simulink model "H_inf_2021"  (R2021b)
settings: Solver=VariableStepAuto  StartTime=0.0  StopTime=20  FixedStep=0.01  RelTol=1e-3
values from neighbouring files (symbols this model uses):
  Ask = [0 1 0 0 ... (first row only)    [H_inf_ctrl.m]    (also in H_inf_ctrl_11_2_p.m; H_inf_ctrl_11_3_heavy.m; H_inf_ctrl_11_3_light.m)
  Bsk = [0 0 0 0 ... (first row only)    [H_inf_ctrl.m]    (also in H_inf_ctrl_11_2_p.m; H_inf_ctrl_11_3_heavy.m; H_inf_ctrl_11_3_light.m)
  Csk = [0 1 0 0 ... (first row only)    [H_inf_ctrl.m]    (also in H_inf_ctrl_11_2_p.m; H_inf_ctrl_11_3_heavy.m; H_inf_ctrl_11_3_light.m)
  Dsk = zeros(2,4)    [H_inf_ctrl.m]    (also in H_inf_ctrl_11_2_p.m; H_inf_ctrl_11_3_heavy.m; H_inf_ctrl_11_3_light.m)
undefined symbols (not defined in the file or in its folder): Ainf, Binf, Cinf, Dinf, sigbuilder_block
settings Model: Creator=tawsiful  LastModifiedBy=rivaa
settings DebuggingCC: UnconnectedInputMsg=none  UnconnectedOutputMsg=none  UnconnectedLineMsg=none
settings RTWCC: DLArmComputeVersion=20.02.1

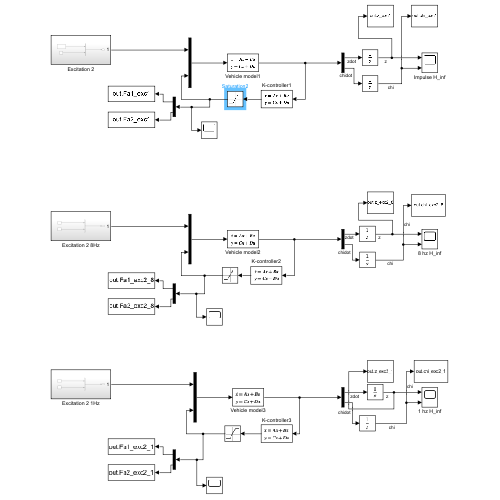
[thumbnail: Simulink's stored preview of the top-level diagram]
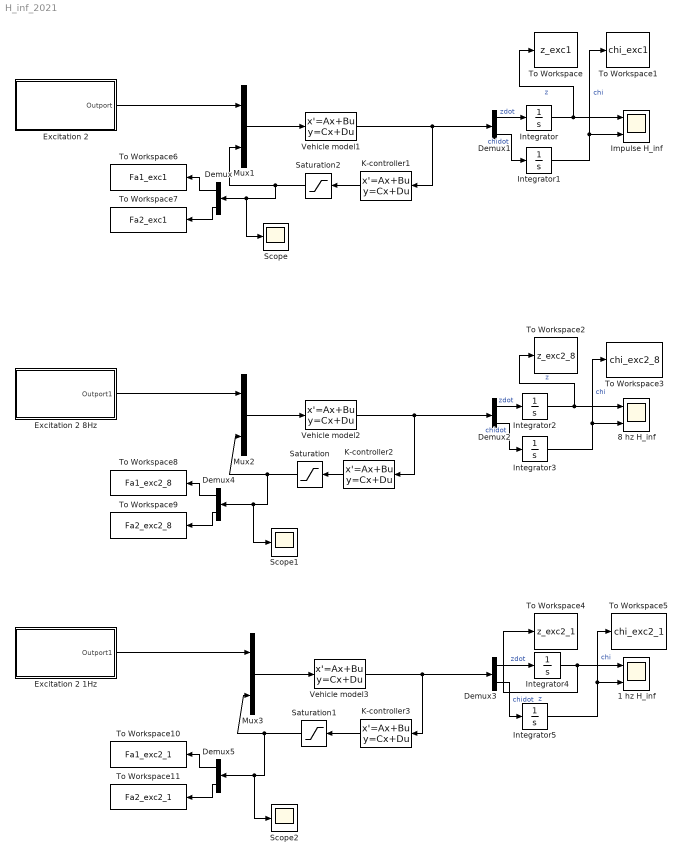
== system H_inf_2021 ==
  1 hz H_inf : Scope  NumInputPorts=2
  8 hz H_inf : Scope  NumInputPorts=2
  Demux{,1..5} (6 alike) : Demux  Outputs=2
  Excitation 2 : Subsystem
  Excitation 2 1Hz : Subsystem
  Excitation 2 8Hz : Subsystem
  Impulse H_inf : Scope  NumInputPorts=2
  Integrator{,1..5} (6 alike) : Integrator
  K-controller1 : StateSpace  A=Ainf  B=Binf  C=Cinf  D=Dinf  InitialCondition=0
  K-controller2 : StateSpace  A=Ainf  B=Binf  C=Cinf  D=Dinf  InitialCondition=0
  K-controller3 : StateSpace  A=Ainf  B=Binf  C=Cinf  D=Dinf  InitialCondition=0
  Mux1 : Mux  Inputs=2
  Mux2 : Mux  Inputs=2
  Mux3 : Mux  Inputs=2
  Saturation : Saturate  UpperLimit=10e3  LowerLimit=-10e3
  Saturation1 : Saturate  UpperLimit=10e3  LowerLimit=-10e3
  Saturation2 : Saturate  UpperLimit=10e3  LowerLimit=-10e3
  Scope : Scope
  Scope1 : Scope
  Scope2 : Scope
  To Workspace : ToWorkspace  VariableName=z_exc1  SampleTime=-1
      settings: Save2DSignal=2-D array (concatenate along first dimension)
  To Workspace1 : ToWorkspace  VariableName=chi_exc1  SampleTime=-1
      settings: Save2DSignal=2-D array (concatenate along first dimension)
  To Workspace10 : ToWorkspace  VariableName=Fa1_exc2_1  SampleTime=-1
  To Workspace11 : ToWorkspace  VariableName=Fa2_exc2_1  SampleTime=-1
  To Workspace2 : ToWorkspace  VariableName=z_exc2_8  SampleTime=-1
      settings: Save2DSignal=2-D array (concatenate along first dimension)
  To Workspace3 : ToWorkspace  VariableName=chi_exc2_8  SampleTime=-1
      settings: Save2DSignal=2-D array (concatenate along first dimension)
  To Workspace4 : ToWorkspace  VariableName=z_exc2_1  SampleTime=-1
      settings: Save2DSignal=2-D array (concatenate along first dimension)
  To Workspace5 : ToWorkspace  VariableName=chi_exc2_1  SampleTime=-1
      settings: Save2DSignal=2-D array (concatenate along first dimension)
  To Workspace6 : ToWorkspace  VariableName=Fa1_exc1  SampleTime=-1
  To Workspace7 : ToWorkspace  VariableName=Fa2_exc1  SampleTime=-1
  To Workspace8 : ToWorkspace  VariableName=Fa1_exc2_8  SampleTime=-1
  To Workspace9 : ToWorkspace  VariableName=Fa2_exc2_8  SampleTime=-1
  Vehicle model1 : StateSpace  A=Ask  B=Bsk  C=Csk  D=Dsk  InitialCondition=0
  Vehicle model2 : StateSpace  A=Ask  B=Bsk  C=Csk  D=Dsk  InitialCondition=0
  Vehicle model3 : StateSpace  A=Ask  B=Bsk  C=Csk  D=Dsk  InitialCondition=0
  wires:
  Demux3/1 -> Integrator4/1  "zdot"
  Demux3/2 -> Integrator5/1  "chidot"
  Demux1/2 -> Integrator1/1  "chidot"
  Demux2/2 -> Integrator3/1  "chidot"
  Demux1/1 -> Integrator/1  "zdot"
  Demux2/1 -> Integrator2/1  "zdot"
  Mux1/1 -> Vehicle model1/1
  Vehicle model1/1 -> Demux1/1, K-controller1/1
  K-controller1/1 -> Saturation2/1
  Vehicle model2/1 -> Demux2/1, K-controller2/1
  Mux2/1 -> Vehicle model2/1
  Mux3/1 -> Vehicle model3/1
  Vehicle model3/1 -> Demux3/1, K-controller3/1
  K-controller3/1 -> Saturation1/1
  Excitation 2/1(Outport) -> Mux1/1
  Excitation 2 8Hz/1(Outport1) -> Mux2/1
  Excitation 2 1Hz/1(Outport1) -> Mux3/1
  Demux/1 -> To Workspace6/1
  Demux/2 -> To Workspace7/1
  Demux4/2 -> To Workspace9/1
  Demux4/1 -> To Workspace8/1
  Demux5/1 -> To Workspace10/1
  Demux5/2 -> To Workspace11/1
  Integrator/1 -> To Workspace/1, Impulse H_inf/1  "z"
  Integrator1/1 -> To Workspace1/1, Impulse H_inf/2  "chi"
  Integrator2/1 -> To Workspace2/1, 8 hz H_inf/1  "z"
  Integrator3/1 -> To Workspace3/1, 8 hz H_inf/2  "chi"
  Integrator4/1 -> To Workspace4/1, 1 hz H_inf/1  "z"
  Integrator5/1 -> To Workspace5/1, 1 hz H_inf/2  "chi"
  K-controller2/1 -> Saturation/1
  Saturation/1 -> Scope1/1, Demux4/1, Mux2/2
  Saturation1/1 -> Scope2/1, Demux5/1, Mux3/2
  Saturation2/1 -> Mux1/2, Scope/1, Demux/1

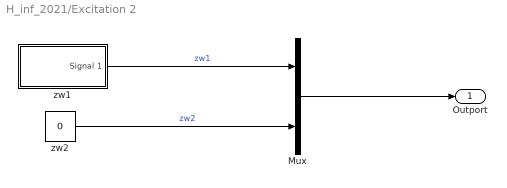
== system H_inf_2021/Excitation 2 ==
  Mux : Mux  Inputs=2
  zw1 : Subsystem  Tag=STV Subsys  LoadFcn=sigbuilder_block('load');  StartFcn=sigbuilder_block('start');  StopFcn=sigbuilder_block('stop');  ClipboardFcn=sigbuilder_block('clipboard');  mask(Sigbuilder block){tuvar=[0:10]}
      mask help: Simulink:masks:SigbuilderBlock_MD
      mask init:
      | if ~strcmp(get_param(bdroot(gcbh),'SimulationStatus'),'stopped') tuvar = sigbuilder_block('maskInit'); end
      settings: CopyFcn=sigbuilder_block('copy');  DeleteFcn=sigbuilder_block('delete');  ModelCloseFcn=sigbuilder_block('modelClose');  PreSaveFcn=sigbuilder_block('preSave');  PauseFcn=sigbuilder_block('pause');  ContinueFcn=sigbuilder_block('continue');  NameChangeFcn=sigbuilder_block('namechange');  OpenFcn=sigbuilder_block('open',[437.6 199.2 550.4 400 ]);  CloseFcn=sigbuilder_block('close');
      mask Display: plot(0, 0, 100, 100,[2, 2, 32, 32, 2], [68, 8, 8, 68, 68],[32, 2], [38, 38], [32, 19, 2],[53, 60, 44], [32, 17, 17, 2],[16, 16, 31, 31]);txt = getActiveGroup(gcbh);text(2, 100, txt,'verticalAlignment', 'top');
  zw2 : Constant  Value=0
  Outport : Outport
  wires:
  zw1/1(Signal 1) -> Mux/1  "zw1"
  zw2/1 -> Mux/2  "zw2"
  Mux/1 -> Outport/1

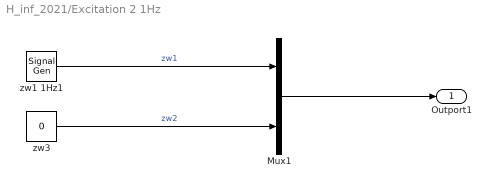
== system H_inf_2021/Excitation 2 1Hz ==
  Mux1 : Mux  Inputs=2
  zw1 1Hz1 : SignalGenerator  Amplitude=0.01  Frequency=2*pi*1  Units=rad/sec
  zw3 : Constant  Value=0
  Outport1 : Outport
  wires:
  zw3/1 -> Mux1/2  "zw2"
  zw1 1Hz1/1 -> Mux1/1  "zw1"
  Mux1/1 -> Outport1/1

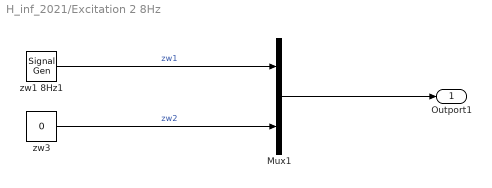
== system H_inf_2021/Excitation 2 8Hz ==
  Mux1 : Mux  Inputs=2
  zw1 8Hz1 : SignalGenerator  Amplitude=0.01  Frequency=2*pi*8  Units=rad/sec
  zw3 : Constant  Value=0
  Outport1 : Outport
  wires:
  zw3/1 -> Mux1/2  "zw2"
  zw1 8Hz1/1 -> Mux1/1  "zw1"
  Mux1/1 -> Outport1/1

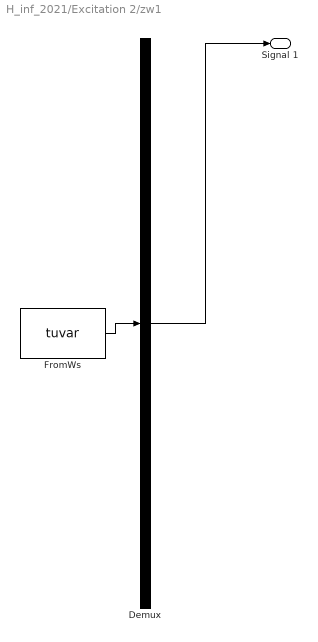
== system H_inf_2021/Excitation 2/zw1 ==
  Demux : Demux  Tag=STV Demux  Outputs=1
      settings: DisplayOption=none
  FromWs : FromWorkspace  Tag=STV FromWs  VariableName=tuvar
      SigBuilderData=|
      | common.afterFinalStr = 'Extrapolate'
      | common.sampleTime = 0
      | dataSet.timeRange = [0 10]
      | dataSet.name = 'Group 1'
      | sbobj.Groups.Name = 'Group 1'
      | sbobj.Groups.Signals.Name = 'Signal 1'
      | sbobj.Groups.Signals.XData = [0 0.1 0.1 10]
      | sbobj.Groups.Signals.YData = [0.03 0.03 0 0]
  Signal 1 : Outport  Tag=STV Outport
  wires:
  Demux/1 -> Signal 1/1
  FromWs/1 -> Demux/1
